simulink model "regen"  (R2025b)
settings: Solver=VariableStepAuto  StartTime=0.0  StopTime=1  RelTol=1e-3
libraries: fuzblock x1
settings Model: Creator=jessi  LastModifiedBy=jessi

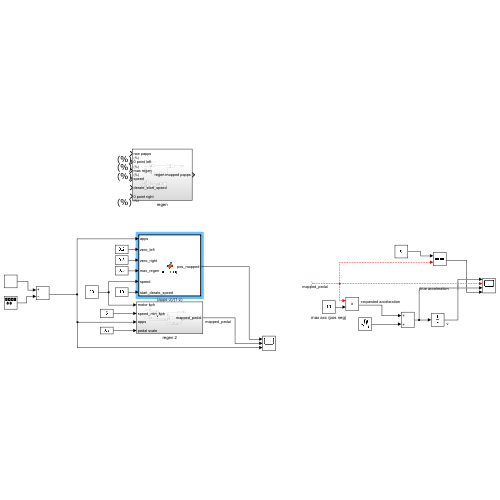
[thumbnail: Simulink's stored preview of the top-level diagram]
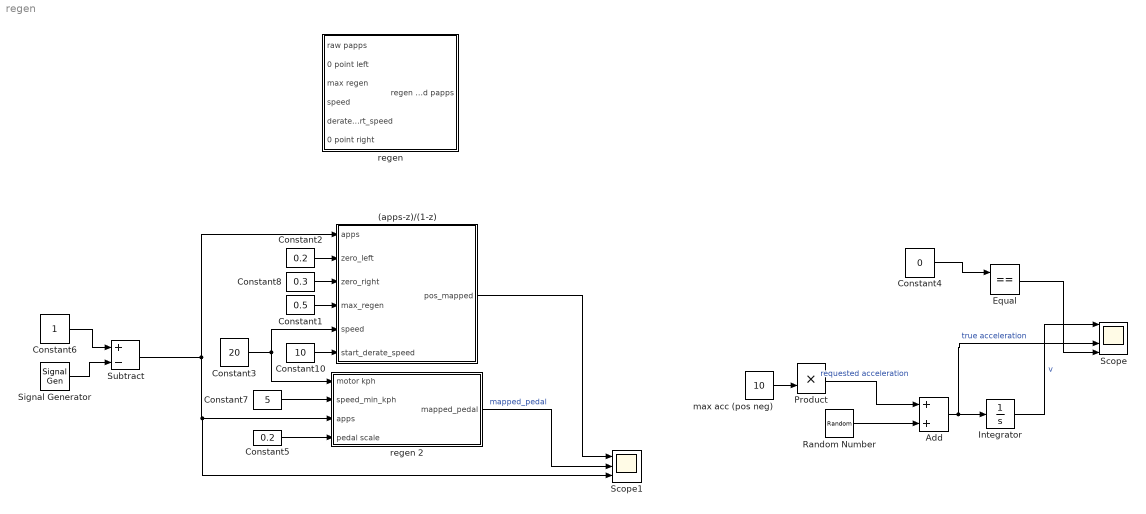
== system regen ==
  (apps-z)/(1-z) : MATLAB Function  TreatAsAtomicUnit=on
  Add : Sum
  Constant1 : Constant  Value=0.5
  Constant10 : Constant  Value=10
  Constant2 : Constant  Value=0.2
  Constant3 : Constant  Value=20
  Constant4 : Constant  Value=0
  Constant5 : Constant  Value=0.2
  Constant6 : Constant
  Constant7 : Constant  Value=5
  Constant8 : Constant  Value=0.3
  Equal : RelationalOperator  Operator===  OutDataTypeStr=boolean  RndMeth=Simplest  InputSameDT=off
  Integrator : Integrator  InitialCondition=20
  Product : Product
  Random Number : RandomNumber  Variance=2  SampleTime=0.01
  Scope : Scope  NumInputPorts=4
      settings: ActiveDisplayYMinimum=19.682739386041991  ActiveDisplayYMaximum=20.456271960293634
  Scope1 : Scope  NumInputPorts=3
      settings: ActiveDisplayYMinimum=-3.497979479536852  ActiveDisplayYMaximum=3.28773480617738  DataLoggingVariableName=ScopeData2
  Signal Generator : SignalGenerator  WaveForm=sawtooth  Frequency=0.99
  Subtract : Sum  Inputs=+-
  max acc (pos neg) : Constant  Value=10
  regen : Subsystem
  regen 2 : Subsystem
  wires:
  Product/1 -> Add/1  "requested acceleration"
  Integrator/1 -> Scope/1  "v"
  max acc (pos neg)/1 -> Product/2
  Signal Generator/1 -> Subtract/2
  Random Number/1 -> Add/2
  Add/1 -> Integrator/1, Scope/3  "true acceleration"
  Constant4/1 -> Equal/1
  Equal/1 -> Scope/4
  Constant5/1 -> regen 2/4(pedal scale)
  ? -> Product/1, Scope/2, Equal/2  "mapped_pedal"
  regen 2/1(mapped_pedal) -> Scope1/2  "mapped_pedal"
  Constant7/1 -> regen 2/2(speed_min_kph)
  Constant6/1 -> Subtract/1
  Subtract/1 -> (apps-z)/(1-z)/1(apps), Scope1/3, regen 2/3(apps)
  Constant1/1 -> (apps-z)/(1-z)/4(max_regen)
  Constant2/1 -> (apps-z)/(1-z)/2(zero_left)
  Constant8/1 -> (apps-z)/(1-z)/3(zero_right)
  Constant3/1 -> regen 2/1(motor kph), (apps-z)/(1-z)/5(speed)
  Constant10/1 -> (apps-z)/(1-z)/6(start_derate_speed)
  (apps-z)/(1-z)/1(pos_mapped) -> Scope1/1

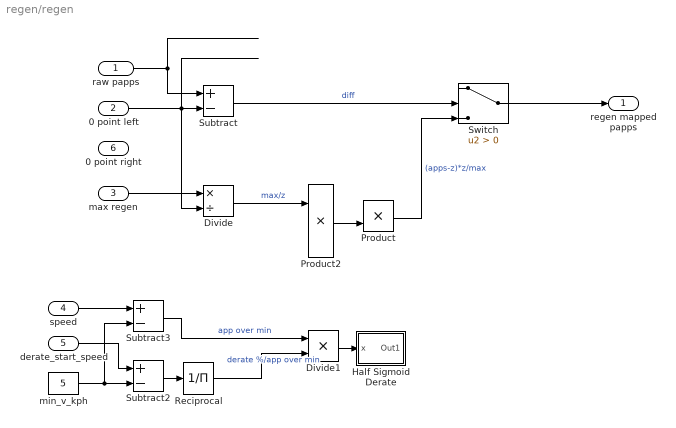
== system regen/regen ==
  raw papps : Inport  Unit=%
  0 point left : Inport  Port=2  Unit=%
  max regen : Inport  Port=3  Unit=%
  speed : Inport  Port=4
  derate_start_speed : Inport  Port=5
  0 point right : Inport  Port=6  Unit=%
  Divide : Product  Inputs=*/
  Divide1 : Product  Inputs=**
  Half Sigmoid Derate : Subsystem
  Product : Product
  Product2 : Product
  Reciprocal : Product  Inputs=/
  Subtract : Sum  Inputs=+-
  Subtract2 : Sum  Inputs=+-
  Subtract3 : Sum  Inputs=+-
  Switch : Switch  Criteria=u2 > Threshold  SaturateOnIntegerOverflow=off  InputSameDT=off
  min_v_kph : Constant  Value=5
  regen mapped papps : Outport
  wires:
  0 point left/1 -> Divide/2, Subtract/2
  Product/1 -> Switch/3  "(apps-z)*z/max"
  Switch/1 -> regen mapped papps/1
  max regen/1 -> Divide/1
  raw papps/1 -> Subtract/1
  Divide/1 -> Product2/1  "max/z"
  derate_start_speed/1 -> Subtract2/1
  Subtract2/1 -> Reciprocal/1
  min_v_kph/1 -> Subtract2/2, Subtract3/2
  speed/1 -> Subtract3/1
  Subtract3/1 -> Divide1/1  "app over min"
  Product2/1 -> Product/2
  Reciprocal/1 -> Divide1/2  "derate %/app over min"
  Divide1/1 -> Half Sigmoid Derate/1(x)
  Subtract/1 -> Switch/2  "diff"
  ? -> Switch/1

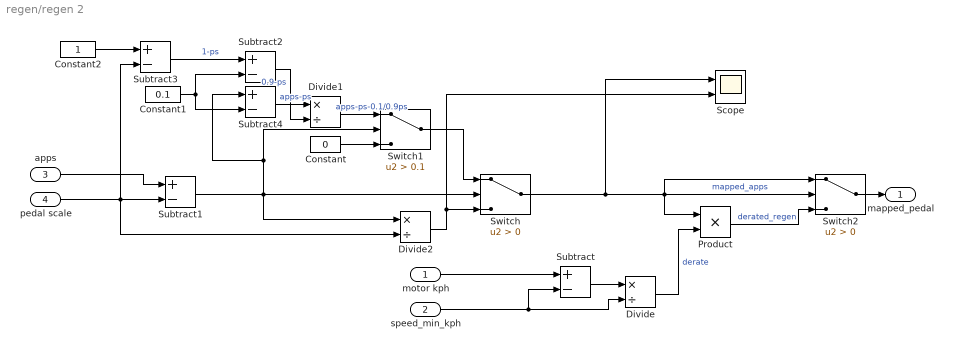
== system regen/regen 2 ==
  motor kph : Inport
  speed_min_kph : Inport  Port=2
  apps : Inport  Port=3
  pedal scale : Inport  Port=4
  Constant : Constant  Value=0
  Constant1 : Constant  Value=0.1
  Constant2 : Constant
  Divide : Product  Inputs=*/
  Divide1 : Product  Inputs=*/
  Divide2 : Product  Inputs=*/
  Product : Product
  Scope : Scope  NumInputPorts=2
      settings: ActiveDisplayYMinimum=-1.1  ActiveDisplayYMaximum=-0.9
  Subtract{,1..4} (5 alike) : Sum  Inputs=+-
  Switch : Switch  Criteria=u2 > Threshold  SaturateOnIntegerOverflow=off  InputSameDT=off
  Switch1 : Switch  Criteria=u2 > Threshold  Threshold=0.1  SaturateOnIntegerOverflow=off  InputSameDT=off
  Switch2 : Switch  Criteria=u2 > Threshold  SaturateOnIntegerOverflow=off  InputSameDT=off
  mapped_pedal : Outport
  wires:
  motor kph/1 -> Subtract/1
  speed_min_kph/1 -> Divide/2, Subtract/2
  Subtract/1 -> Divide/1
  apps/1 -> Subtract1/1
  pedal scale/1 -> Divide2/2, Subtract1/2, Subtract3/2
  Subtract1/1 -> Divide2/1, Switch/2, Switch1/2, Subtract4/1
  Switch1/1 -> Switch/1
  Constant/1 -> Switch1/3
  Constant1/1 -> Subtract4/2, Subtract2/2
  Constant2/1 -> Subtract3/1
  Subtract3/1 -> Subtract2/1  "1-ps"
  Subtract2/1 -> Divide1/2  "0.9-ps"
  Subtract4/1 -> Divide1/1  "apps-ps"
  Divide1/1 -> Switch1/1  "apps-ps-0.1/0.9ps"
  Divide2/1 -> Switch/3, Scope/2
  Switch/1 -> Switch2/1, Switch2/2, Product/1, Scope/1  "mapped_apps"
  Divide/1 -> Product/2  "derate"
  Switch2/1 -> mapped_pedal/1
  Product/1 -> Switch2/3  "derated_regen"

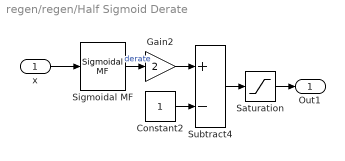
== system regen/regen/Half Sigmoid Derate ==
  x : Inport
  Constant2 : Constant
  Gain2 : Gain  Gain=2
  Saturation : Saturate  UpperLimit=1  LowerLimit=0
  Sigmoidal MF : fuzblock/Membership  Functions/Sigmoidal MF  a=3  c=0
  Subtract4 : Sum  Inputs=+-
  Out1 : Outport
  wires:
  Subtract4/1 -> Saturation/1
  Sigmoidal MF/1 -> Gain2/1  "derate"
  Saturation/1 -> Out1/1
  Constant2/1 -> Subtract4/2
  x/1 -> Sigmoidal MF/1
  Gain2/1 -> Subtract4/1

== matlab function regen/(apps-z)//(1-z) ==
  data: apps input; pos_mapped output; zero_left input; zero_right input; max_regen input; speed input; start_derate_speed input
function pos_mapped = pos_map(apps, zero_left, zero_right, max_regen, speed, start_derate_speed)
    if apps < zero_left
        % regen condition
        unclipped_derate_term = (speed - 5)/(start_derate_speed - 5);
        derate_term = max(0, min(1, unclipped_derate_term));
        pos_mapped = (apps - zero_left) / zero_left * max_regen * derate_term;
    elseif zero_left <= apps && apps <= zero_right
        pos_mapped = 0;
    else % apps > zero_right
        pos_mapped = (apps-zero_right)/(1-zero_right);
    end
end
